simulink model "reaction_pendulum_LQR_LETSEEWHATHAPPENSGUYS"  (R2021b)
settings: Solver=FixedStepDiscrete  StartTime=0.0  StopTime=inf  FixedStep=h  RelTol=1e-3  EnableMultiTasking=on
PreLoadFcn:
  | warning('off','MATLAB:dispatcher:InexactMatch');
InitFcn:
  | hwinit
values from neighbouring files (symbols this model uses):
  A = [0.989609173212  0  0; 0  1  0.01; -0.000301949872013  -0.0950246262215  0.997224421049]    [MATRICES.mat]    (also in SS_11_5.mat = [0.9904  0  0; 0  1  0.01; -9e-05  -0.033262024  0.99812133]; WEAREGOINGHOMEMATRICES.mat = [0.989609173212  0  0; 0  1  0.01; 0.000423899858033  -0.095; current_SS.mat = [0.989609173212  0  0; 0  1  0.01; -9.34612180115e-05  -0.02; dynamicUpdateModel.m = [1.000494318995348 0.010001647563961 2.391143629140888e-07)
  Aeq = [Aeq; Ax0]    [Manual_MPC_Companion.m]    (also in Manual_MPC_Companion_THURSDAY.m = zeros(n * Np, n_total))
  B = [4.20519003073 0 0]    [MATRICES.mat]    (also in SS_11_5.mat = [4.1334 0 0]; current_SS.mat; dynamicUpdateModel.m = [-1.828407620987413e-04; full_dynamics.m = dsys.B)
  beq = zeros(n_total,1)    [Manual_MPC_Companion.m]    (also in Manual_MPC_Companion_THURSDAY.m = zeros(n * Np, 1))
  C = [1 0 0; 0 1 0]    [MeasModel.m]    (also in SS_11_5.mat = [1  0  0; 0  1  0]; current_SS.mat = [1  0  0; 0  1  0]; full_dynamics.m = dsys.C; full_system_ID.m = sys_est.C)
  H = diag([kron(ones(1,Np), Q) kron(ones(1,Np), R)])    [Manual_MPC_Companion.m]    (also in Manual_MPC_Companion_THURSDAY.m = blkdiag(Qbar, Rbar))
  h = 0.01    [SS_11_5.mat]    (also in hwinit.m)
  lb = [-1e6*ones(nx_total,1); -ones(m*Np,1)]    [Manual_MPC_Companion.m]    (also in Manual_MPC_Companion_THURSDAY.m = [-1e6*ones(nx_total, 1); -ones(nu_total, 1)])
  ub = [1e6*ones(nx_total,1); ones(m*Np,1)]    [Manual_MPC_Companion.m]    (also in Manual_MPC_Companion_THURSDAY.m = [ 1e6*ones(nx_total, 1);  ones(nu_total, 1)])
undefined symbols (not defined in the file or in its folder): cThresh, Discrete, E_ref, g_eff, K, K_bottom, k_e, magnitude, Time
libraries: simulink x3, ctrlSharedLib x2, mpclib x1
settings Model: SimulationMode=external  ExtModeTrigDuration=100000  Creator=user  LastModifiedBy=suray
settings DataIOCC: SaveFormat=Array  SignalLoggingSaveFormat=ModelDataLogs  SaveOutput=off  SignalLogging=off  DSMLogging=off  SaveTime=off  ReturnWorkspaceOutputs=off
settings OptimizationCC: ExpressionDepthLimit=2147483647  LifeSpan=inf
settings DebuggingCC: UnderspecifiedInitializationDetection=Classic  MergeDetectMultiDrivingBlocksExec=none  SolverPrmCheckMsg=warning  FcnCallInpInsideContextMsg=warning  StateNameClashWarn=warning  SFUnexpectedBacktrackingDiag=warning  SFNoUnconditionalDefaultTransitionDiag=warning  SFExecutionAtInitializationDiag=none  ArithmeticOperatorsInVariantConditions=warning
settings HardwareCC: ProdBitPerPointer=32  ProdBitPerSizeT=32  ProdBitPerPtrDiffT=32  ProdLargestAtomicFloat=None  ProdIntDivRoundTo=Undefined  ProdEndianess=Unspecified  ProdWordSize=32  ProdHWDeviceType=32-bit Generic
settings ModelReferenceCC: PropagateSignalLabelsOutOfModel=off
settings SFSimCC: SimUseLocalCustomCode=off  CustomCodeUndefinedFunction=UseInterfaceOnly
settings RTWCC: Description=rpend RTDAC/USB2 (Visual C/C++)  SystemTargetFile=rtcon_rpend_usb2.tlc  TemplateMakefile=rtcon_rpend_vc_usb2_x64.tmf  RTWUseLocalCustomCode=off
settings CodeAppCC: StateflowObjectComments=on
settings STFCustomTargetCC: ModelReferenceCompliant=off  CombineOutputUpdateFcns=on  MatFileLogging=on  GRTInterface=off  SystemTargetFile=rtcon_rpend_usb2.tlc
settings GRTTargetCC: TargetLangStandard=C89/C90 (ANSI)  ModelReferenceCompliant=off  ParMdlRefBuildCompliant=off  CompOptLevelCompliant=off  ConcurrentExecutionCompliant=off  CPPClassGenCompliant=off  UseToolchainInfoCompliant=off  ExtMode=on  ExtModeMexFile=rtcon_ext_comm
settings ConfigComp: CovMetricSettings=dw  CovSaveCumulativeToWorkspaceVar=on  CovSaveSingleToWorkspaceVar=on  CovExternalEMLEnable=off  CovSFcnEnable=off

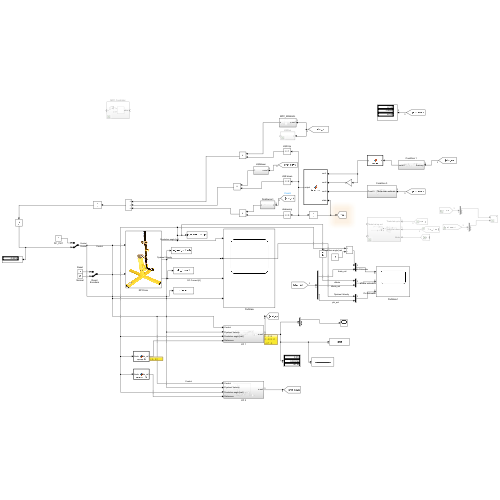
[thumbnail: Simulink's stored preview of the top-level diagram]
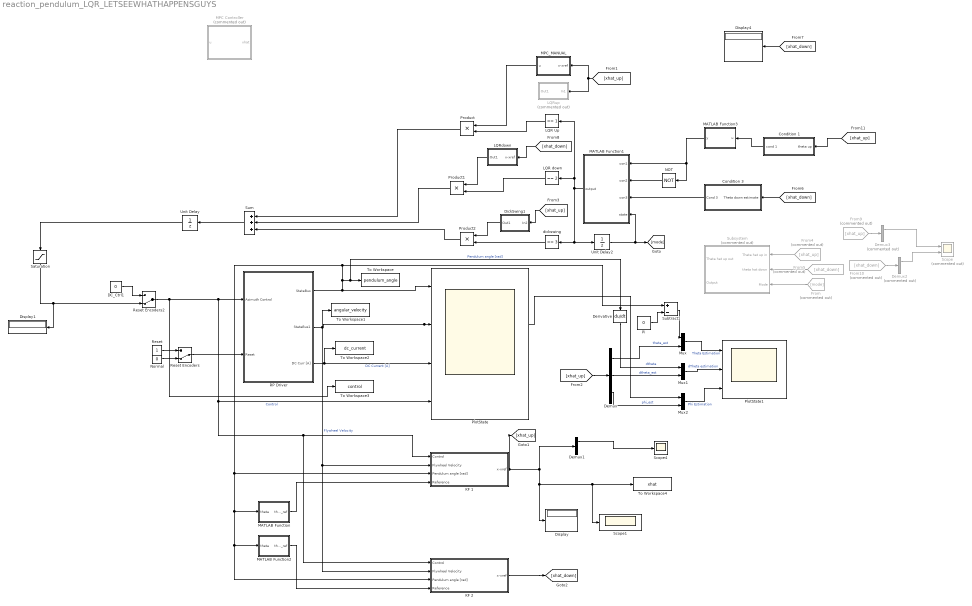
== system reaction_pendulum_LQR_LETSEEWHATHAPPENSGUYS ==
  Condition 1 : Subsystem
  Condition 3 : Subsystem
  DC_Ctrl1 : Constant  Value=0
  Demux : Demux  Outputs=3
  Demux1 : Demux  Outputs=3
  Demux2 : Demux  Commented=on  Outputs=3
  Demux3 : Demux  Commented=on  Outputs=3
  Derivative : Derivative
  DickSwing1 : Subsystem
  Display : Display
  Display1 : Display
  Display4 : Display
  From : From  Commented=on  GotoTag=mode
  From10 : From  Commented=on  GotoTag=xhat_down
  From4 : From  Commented=on  GotoTag=xhat_up
  From5 : From  Commented=on  GotoTag=xhat_down
  From9 : From  Commented=on  GotoTag=xhat_up
  KF 1 : Subsystem
  KF 2 : Subsystem
  LQR Up : simulink/Logic and Bit Operations/Compare To Constant  relop===  const=1  OutDataTypeStr=uint8
  LQR down : simulink/Logic and Bit Operations/Compare To Constant  relop===  const=2  OutDataTypeStr=uint8
  LQRdown : Subsystem
  LQRup : Subsystem  Commented=on
  MATLAB Function : MATLAB Function  TreatAsAtomicUnit=on
  MATLAB Function1 : MATLAB Function  TreatAsAtomicUnit=on
  MATLAB Function2 : MATLAB Function  TreatAsAtomicUnit=on
  MATLAB Function3 : MATLAB Function  TreatAsAtomicUnit=on
  MPC Controller : Subsystem  Commented=on
  MPC_MANUAL : Subsystem
  Mux : Mux  Inputs=2
  Mux1 : Mux  Inputs=2
  Mux2 : Mux  Inputs=2
  NOT : Logic  Operator=NOT  IconShape=distinctive  AllPortsSameDT=off  OutDataTypeStr=boolean
  Normal : Constant  Value=0
  Pi : Constant  Value=0  OutDataTypeStr=Inherit: Inherit via back propagation
  PlotState : Scope  NumInputPorts=4
  PlotState1 : Scope  NumInputPorts=3
  Product : Product
  Product1 : Product
  Product2 : Product
  RP Driver : Subsystem
      mask Display: image(imread('rwp.JPG'))
  Reset : Constant
  Reset Encoders : ManualSwitch  CurrentSetting=0
  Reset Encoders2 : ManualSwitch  CurrentSetting=0
  Saturation : Saturate  UpperLimit=1  LowerLimit=-1
  Scope : Scope  Commented=on  NumInputPorts=2
  Scope1 : Scope
  Scope4 : Scope
  Subsystem : Subsystem  Commented=on
  Subtract1 : Sum  Inputs=+-
  Sum : Sum  Inputs=+++
  To Workspace : ToWorkspace  VariableName=pendulum_angle  SaveFormat=Timeseries  SampleTime=-1
  To Workspace1 : ToWorkspace  VariableName=angular_velocity  SaveFormat=Timeseries  SampleTime=-1
  To Workspace2 : ToWorkspace  VariableName=dc_current  SaveFormat=Timeseries  SampleTime=-1
  To Workspace3 : ToWorkspace  VariableName=control  SaveFormat=Timeseries  SampleTime=-1
  To Workspace4 : ToWorkspace  VariableName=xhat  SaveFormat=Timeseries  SampleTime=-1
  Unit Delay : UnitDelay  SampleTime=0.01
  Unit Delay2 : UnitDelay  InitialCondition=3  SampleTime=h  HasFrameUpgradeWarning=on
  dickswing : simulink/Logic and Bit Operations/Compare To Constant  relop===  const=3  OutDataTypeStr=uint8
  wires:
  Normal/1 -> Reset Encoders/2
  Reset/1 -> Reset Encoders/1
  Reset Encoders/1 -> RP Driver/2(Reset)
  RP Driver/3(DC Curr [A]) -> To Workspace2/1, PlotState/3  "DC Current [A]"
  RP Driver/1(StateBus) -> Derivative/1, To Workspace/1, KF 1/3(Pendulum angle [rad]), KF 2/3(Pendulum angle [rad]), MATLAB Function2/1(theta), MATLAB Function/1(theta), Subtract1/1, PlotState/1  "Pendulum angle [rad]"
  Demux/3 -> Mux2/2  "phi_est"
  Demux/2 -> Mux1/2  "dtheta_est"
  Demux/1 -> Mux/2  "theta_est"
  Derivative/1 -> Mux1/1  "dtheta"
  Mux/1 -> PlotState1/1  "Theta Estimation"
  Mux1/1 -> PlotState1/2  "dTheta estimation"
  Mux2/1 -> PlotState1/3  "Phi Estimation"
  Saturation/1 -> Display1/1, Reset Encoders2/2
  DC_Ctrl1/1 -> Reset Encoders2/1
  Pi/1 -> Subtract1/2
  Subtract1/1 -> Mux/1
  Unit Delay/1 -> Saturation/1
  Unit Delay2/1 -> MATLAB Function1/4(state), [mode]
  LQR Up/1 -> Product/2
  LQR down/1 -> Product1/2
  MATLAB Function1/1(output) -> dickswing/1, Unit Delay2/1, LQR Up/1, LQR down/1
  dickswing/1 -> Product2/2
  Product/1 -> Sum/1
  Product1/1 -> Sum/2
  Product2/1 -> Sum/3
  NOT/1 -> MATLAB Function1/2(con2)
  DickSwing1/1(Out1) -> Product2/1
  LQRdown/1(Out1) -> Product1/1
  Reset Encoders2/1 -> KF 1/1(Control), KF 2/1(Control), PlotState/4, RP Driver/1(Azimuth Control), To Workspace3/1  "Control"
  RP Driver/2(StateBus1) -> Mux2/1, PlotState/2, To Workspace1/1, KF 2/2(Flywheel Velocity), KF 1/2(Flywheel Velocity)  "Flywheel Velocity"
  MATLAB Function2/1(theta_ref) -> KF 2/4(Reference)
  MATLAB Function/1(theta_ref) -> KF 1/4(Reference)
  KF 2/1(x-xref) -> [xhat_down]
  Sum/1 -> Unit Delay/1
  Demux1/1 -> Scope4/1
  KF 1/1(x-xref) -> [xhat_up], Display/1, Scope1/1, To Workspace4/1, Demux1/1
  From/1 -> Subsystem/3(Mode)
  Condition 3/1(Cond 3) -> MATLAB Function1/3(con3)
  Condition 1/1(cond 1) -> MATLAB Function3/1(u)
  [xhat_up] -> MPC_MANUAL/1(x-xref), LQRup/1(In1)
  [xhat_up] -> Demux/1
  [xhat_up] -> DickSwing1/1(In2)
  From4/1 -> Subsystem/1(Theta hat up in)
  From5/1 -> Subsystem/2(theta hat down)
  [xhat_down] -> Condition 3/1(Theta down estimate)
  [xhat_down] -> Display4/1
  [xhat_down] -> LQRdown/1(x-xref)
  From9/1 -> Demux3/1
  Demux3/1 -> Scope/1
  From10/1 -> Demux2/1
  Demux2/1 -> Scope/2
  MATLAB Function3/1(y) -> MATLAB Function1/1(con1), NOT/1
  [xhat_up] -> Condition 1/1(theta up)
  MPC_MANUAL/1(u) -> Product/1

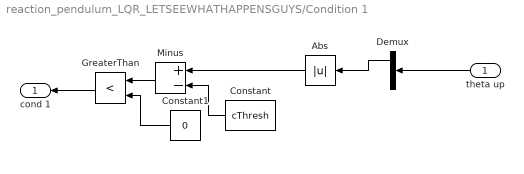
== system reaction_pendulum_LQR_LETSEEWHATHAPPENSGUYS/Condition 1 ==
  theta up : Inport
  Abs : Abs
  Constant : Constant  Value=cThresh
  Constant1 : Constant  Value=0
  Demux : Demux  Outputs=3
  GreaterThan : RelationalOperator  Operator=<  OutDataTypeStr=boolean  RndMeth=Simplest
  Minus : Sum  Inputs=+-
  cond 1 : Outport
  wires:
  Constant1/1 -> GreaterThan/2
  theta up/1 -> Demux/1
  Constant/1 -> Minus/2
  Minus/1 -> GreaterThan/1
  GreaterThan/1 -> cond 1/1
  Abs/1 -> Minus/1
  Demux/1 -> Abs/1

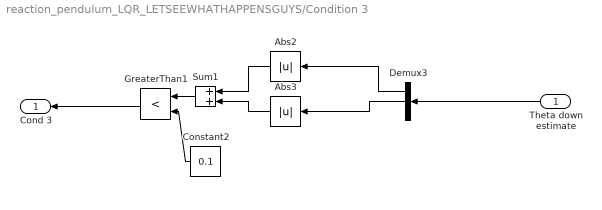
== system reaction_pendulum_LQR_LETSEEWHATHAPPENSGUYS/Condition 3 ==
  Theta down estimate : Inport
  Abs2 : Abs
  Abs3 : Abs
  Constant2 : Constant  Value=0.1
  Demux3 : Demux  Outputs=3
  GreaterThan1 : RelationalOperator  Operator=<  OutDataTypeStr=boolean  RndMeth=Simplest
  Sum1 : Sum
  Cond 3 : Outport
  wires:
  Demux3/2 -> Abs3/1
  Demux3/1 -> Abs2/1
  Abs2/1 -> Sum1/1
  GreaterThan1/1 -> Cond 3/1
  Constant2/1 -> GreaterThan1/2
  Sum1/1 -> GreaterThan1/1
  Abs3/1 -> Sum1/2
  Theta down estimate/1 -> Demux3/1

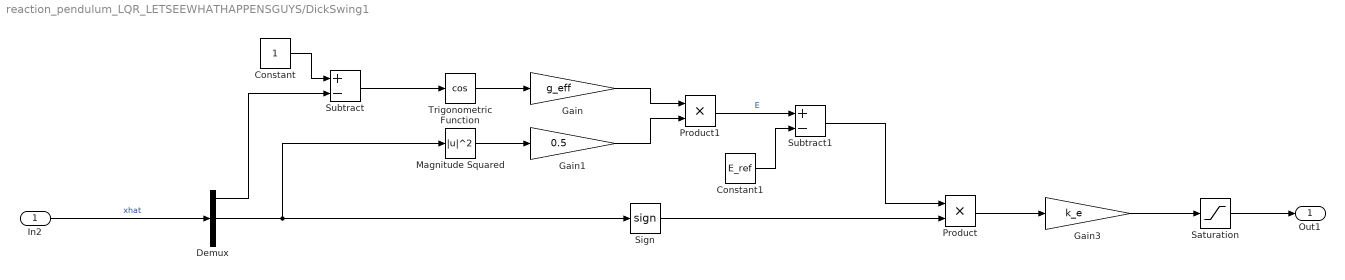
== system reaction_pendulum_LQR_LETSEEWHATHAPPENSGUYS/DickSwing1 ==
  In2 : Inport
  Constant : Constant
  Constant1 : Constant  Value=E_ref
  Demux : Demux  Outputs=3
  Gain : Gain  Gain=g_eff
  Gain1 : Gain  Gain=0.5
  Gain3 : Gain  Gain=k_e
  Magnitude Squared : Math  Operator=magnitude^2  SaturateOnIntegerOverflow=on
  Product : Product
  Product1 : Product
  Saturation : Saturate  UpperLimit=0.75  LowerLimit=-0.75
  Sign : Signum
  Subtract : Sum  Inputs=+-
  Subtract1 : Sum  Inputs=+-
  Trigonometric Function : Trigonometry  Operator=cos
  Out1 : Outport
  wires:
  In2/1 -> Demux/1  "xhat"
  Trigonometric Function/1 -> Gain/1
  Magnitude Squared/1 -> Gain1/1
  Gain/1 -> Product1/1
  Gain1/1 -> Product1/2
  Constant/1 -> Subtract/1
  Subtract/1 -> Trigonometric Function/1
  Demux/1 -> Subtract/2
  Sign/1 -> Product/2
  Product1/1 -> Subtract1/1  "E"
  Constant1/1 -> Subtract1/2
  Subtract1/1 -> Product/1
  Product/1 -> Gain3/1
  Gain3/1 -> Saturation/1
  Demux/2 -> Magnitude Squared/1, Sign/1
  Saturation/1 -> Out1/1

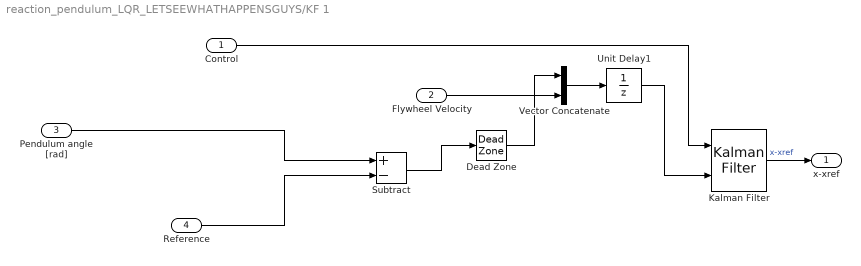
== system reaction_pendulum_LQR_LETSEEWHATHAPPENSGUYS/KF 1 ==
  Control : Inport
  Flywheel Velocity : Inport  Port=2
  Pendulum angle [rad] : Inport  Port=3
  Reference : Inport  Port=4
  Dead Zone : DeadZone  LowerValue=0  UpperValue=0.0  SaturateOnIntegerOverflow=on
  Kalman Filter : ctrlSharedLib/Kalman Filter  TimeDomain=Discrete-Time  UseCurrentEstimator=on  ModelSource=Individual A, B, C, D matrices  ModelSourceVariable=ss(0.95,1,1,0,1)  A=A  B=B  C=C  D=[0;0]  NumberOfStates=1  NumberOfInputs=1  NumberOfOutputs=1  InitialEstimateSource=Dialog  X0=0  P0=10  UseK=off  UseGH=off  NumberOfProcessNoiseInputs=1  G=1  TimeInvariantG=on  H=0  TimeInvariantH=on  Q=diag([0.00001 0.05 0.0001])  TimeInvariantQ=on  R=diag([0.0001 0.01])  TimeInvariantR=on  N=0  TimeInvariantN=on  AddInputPort=on  AddEnablePort=off  OutputEstimatedY=off  OutputP=off  Ts=-1
  Subtract : Sum  Inputs=+-
  Unit Delay1 : UnitDelay  SampleTime=0.01
  Vector Concatenate : Concatenate
  x-xref : Outport
  wires:
  Kalman Filter/1 -> x-xref/1  "x-xref"
  Subtract/1 -> Dead Zone/1
  Reference/1 -> Subtract/2
  Dead Zone/1 -> Vector Concatenate/1
  Flywheel Velocity/1 -> Vector Concatenate/2
  Unit Delay1/1 -> Kalman Filter/2
  Vector Concatenate/1 -> Unit Delay1/1
  Pendulum angle [rad]/1 -> Subtract/1
  Control/1 -> Kalman Filter/1

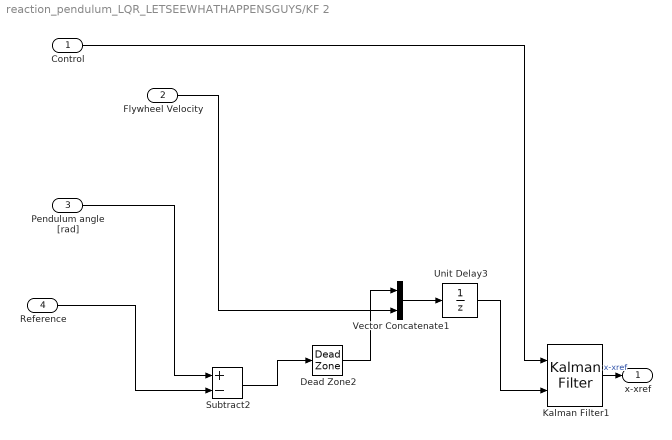
== system reaction_pendulum_LQR_LETSEEWHATHAPPENSGUYS/KF 2 ==
  Control : Inport
  Flywheel Velocity : Inport  Port=2
  Pendulum angle [rad] : Inport  Port=3
  Reference : Inport  Port=4
  Dead Zone2 : DeadZone  LowerValue=0  UpperValue=0.0  SaturateOnIntegerOverflow=on
  Kalman Filter1 : ctrlSharedLib/Kalman Filter  TimeDomain=Discrete-Time  UseCurrentEstimator=on  ModelSource=Individual A, B, C, D matrices  ModelSourceVariable=ss(0.95,1,1,0,1)  A=A  B=B  C=C  D=[0;0]  NumberOfStates=1  NumberOfInputs=1  NumberOfOutputs=1  InitialEstimateSource=Dialog  X0=0  P0=10  UseK=off  UseGH=off  NumberOfProcessNoiseInputs=1  G=1  TimeInvariantG=on  H=0  TimeInvariantH=on  Q=diag([0.00001 0.05 0.0001])  TimeInvariantQ=on  R=diag([0.0001 0.01])  TimeInvariantR=on  N=0  TimeInvariantN=on  AddInputPort=on  AddEnablePort=off  OutputEstimatedY=off  OutputP=off  Ts=-1
  Subtract2 : Sum  Inputs=+-
  Unit Delay3 : UnitDelay  SampleTime=0.01
  Vector Concatenate1 : Concatenate
  x-xref : Outport
  wires:
  Unit Delay3/1 -> Kalman Filter1/2
  Pendulum angle [rad]/1 -> Subtract2/1
  Reference/1 -> Subtract2/2
  Dead Zone2/1 -> Vector Concatenate1/1
  Control/1 -> Kalman Filter1/1
  Subtract2/1 -> Dead Zone2/1
  Vector Concatenate1/1 -> Unit Delay3/1
  Flywheel Velocity/1 -> Vector Concatenate1/2
  Kalman Filter1/1 -> x-xref/1  "x-xref"

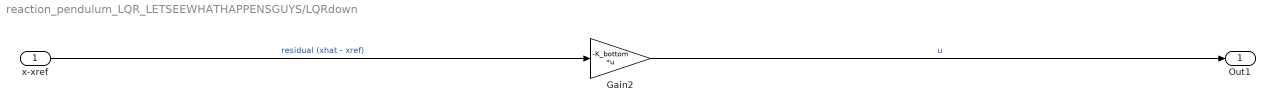
== system reaction_pendulum_LQR_LETSEEWHATHAPPENSGUYS/LQRdown ==
  x-xref : Inport
  Gain2 : Gain  Gain=-K_bottom  Multiplication=Matrix(K*u) (u vector)
  Out1 : Outport
  wires:
  x-xref/1 -> Gain2/1  "residual (xhat - xref)"
  Gain2/1 -> Out1/1  "u"

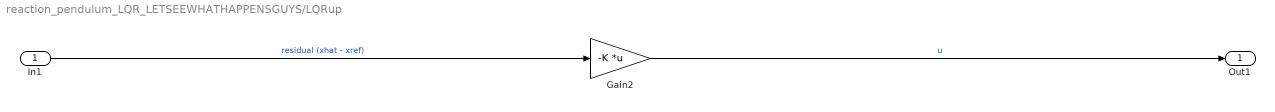
== system reaction_pendulum_LQR_LETSEEWHATHAPPENSGUYS/LQRup ==
  In1 : Inport
  Gain2 : Gain  Gain=-K  Multiplication=Matrix(K*u) (u vector)
  Out1 : Outport
  wires:
  In1/1 -> Gain2/1  "residual (xhat - xref)"
  Gain2/1 -> Out1/1  "u"

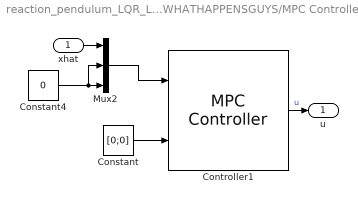
== system reaction_pendulum_LQR_LETSEEWHATHAPPENSGUYS/MPC Controller ==
  xhat : Inport
  Constant : Constant  Value=[0;0]
  Constant4 : Constant  Value=0
  Controller1 : mpclib/MPC Controller  SCDEnableBlockLinearizationSpecification=on  mpcobj=MPC_controller  is_multiple=0  enable_value=0  return_u0=off  updateMPCinCallerWorkspace=on  md_inport=off  mv_inport=off  uref_inport=off  return_cost=off  return_mvseq=off  return_qpstatus=off  return_xseq=off  return_state=off  return_ovseq=off  state_inport=on  umin_inport=off  umax_inport=off  ymin_inport=off  ymax_inport=off  cc_inport=off  ywt_inport=off  uwt_inport=off  duwt_inport=off  rhoeps_inport=off  pm_inport=off  MaximumP=10  HorizonChoice=FixedHorizon  n_ts=0.01  n_p=30  n_mv=1  n_md=0  n_ud=0  n_mo=2  n_uo=0  BlockDataType=double  SampleTimeInherited=off  switch_inport=off
  Mux2 : Mux  Inputs=3
  u : Outport
  wires:
  Controller1/1 -> u/1  "u"
  xhat/1 -> Mux2/1
  Constant4/1 -> Mux2/3, Mux2/2
  Mux2/1 -> Controller1/1
  Constant/1 -> Controller1/2

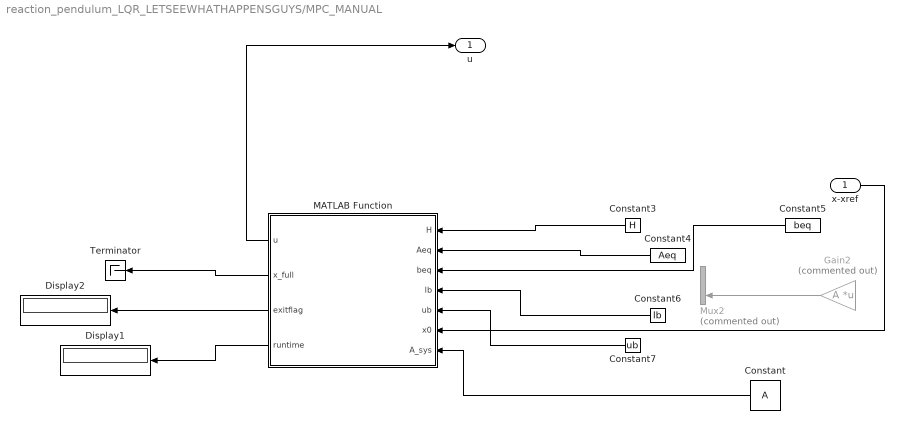
== system reaction_pendulum_LQR_LETSEEWHATHAPPENSGUYS/MPC_MANUAL ==
  x-xref : Inport
  Constant : Constant  Value=A  VectorParams1D=off
  Constant3 : Constant  Value=H
  Constant4 : Constant  Value=Aeq
  Constant5 : Constant  Value=beq
  Constant6 : Constant  Value=lb
  Constant7 : Constant  Value=ub
  Display1 : Display
  Display2 : Display
  Gain2 : Gain  Commented=on  Gain=A  Multiplication=Matrix(K*u) (u vector)
  MATLAB Function : MATLAB Function  TreatAsAtomicUnit=on
  Mux2 : Mux  Commented=on  Inputs=2
  Terminator : Terminator
  u : Outport
  wires:
  Constant3/1 -> MATLAB Function/1(H)
  Constant4/1 -> MATLAB Function/2(Aeq)
  Constant5/1 -> MATLAB Function/3(beq)
  Constant6/1 -> MATLAB Function/4(lb)
  MATLAB Function/3(exitflag) -> Display2/1
  Gain2/1 -> Mux2/2
  Constant7/1 -> MATLAB Function/5(ub)
  MATLAB Function/4(runtime) -> Display1/1
  MATLAB Function/2(x_full) -> Terminator/1
  x-xref/1 -> MATLAB Function/6(x0)
  MATLAB Function/1(u) -> u/1
  Constant/1 -> MATLAB Function/7(A_sys)

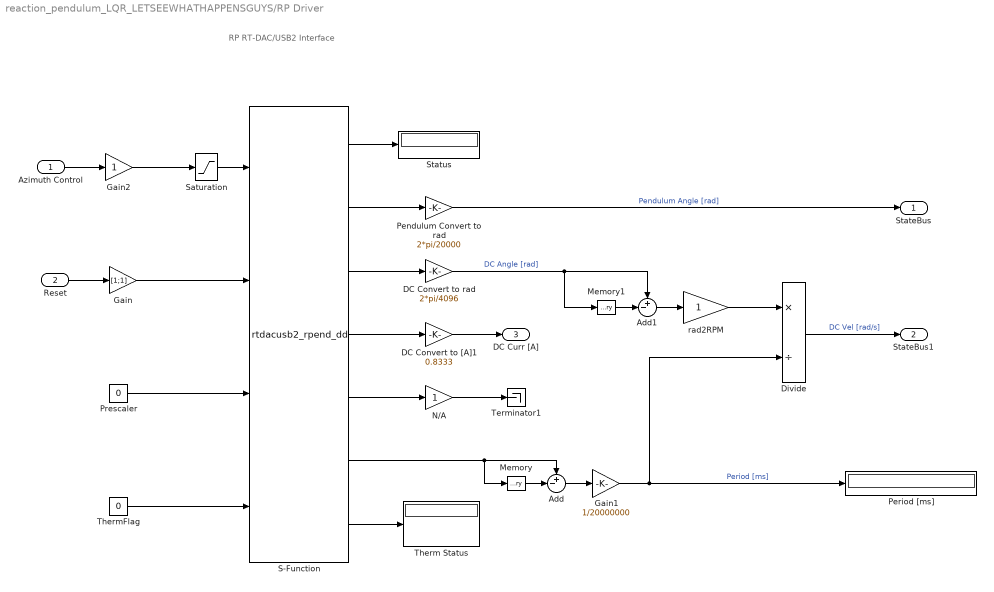
== system reaction_pendulum_LQR_LETSEEWHATHAPPENSGUYS/RP Driver ==
  note: RP RT-DAC/USB2
      | Interface
  Azimuth Control : Inport
  Reset : Inport  Port=2
  Add : Sum  Inputs=+-|
  Add1 : Sum  Inputs=+-|
  DC Convert to [A]1 : Gain  Gain=0.8333  SaturateOnIntegerOverflow=on  OutDataTypeStr=Inherit: Same as input  ParamDataTypeStr=Inherit: Same as input
  DC Convert to rad : Gain  Gain=2*pi/4096  SaturateOnIntegerOverflow=on  OutDataTypeStr=Inherit: Same as input  ParamDataTypeStr=Inherit: Same as input
  Divide : Product  Inputs=*/
  Gain : Gain  Gain=[1;1]
  Gain1 : Gain  Gain=1/20000000
  Gain2 : Gain
  Memory : Memory
  Memory1 : Memory
  N/A : Gain  SaturateOnIntegerOverflow=on  OutDataTypeStr=Inherit: Same as input  ParamDataTypeStr=Inherit: Same as input
  Pendulum Convert to rad : Gain  Gain=2*pi/20000  SaturateOnIntegerOverflow=on  OutDataTypeStr=Inherit: Same as input  ParamDataTypeStr=Inherit: Same as input
  Period [ms] : Display
  Prescaler : Constant  Value=0
  S-Function : S-Function  FunctionName=rtdacusb2_rpend_dd  Parameters=1, h  SFunctionDeploymentMode=off  EnableBusSupport=off
  Saturation : Saturate  UpperLimit=1  LowerLimit=-1
  Status : Display
  Terminator1 : Terminator
  Therm Status : Display
  ThermFlag : Constant  Value=0
  rad2RPM : Gain  SaturateOnIntegerOverflow=on  OutDataTypeStr=Inherit: Same as input  ParamDataTypeStr=Inherit: Same as input
  StateBus : Outport  VectorParamsAs1DForOutWhenUnconnected=off
  StateBus1 : Outport  Port=2  VectorParamsAs1DForOutWhenUnconnected=off
  DC Curr [A] : Outport  Port=3  VectorParamsAs1DForOutWhenUnconnected=off
  wires:
  S-Function/7 -> Therm Status/1
  S-Function/5 -> N/A/1
  S-Function/4 -> DC Convert to [A]1/1
  ThermFlag/1 -> S-Function/4
  Prescaler/1 -> S-Function/3
  Gain/1 -> S-Function/2
  DC Convert to [A]1/1 -> DC Curr [A]/1
  Divide/1 -> StateBus1/1  "DC Vel [rad/s]"
  rad2RPM/1 -> Divide/1
  Add1/1 -> rad2RPM/1
  Memory1/1 -> Add1/2
  N/A/1 -> Terminator1/1
  S-Function/6 -> Add/1, Memory/1
  Gain2/1 -> Saturation/1
  Gain1/1 -> Period [ms]/1, Divide/2  "Period [ms]"
  Add/1 -> Gain1/1
  Memory/1 -> Add/2
  DC Convert to rad/1 -> Add1/1, Memory1/1  "DC Angle [rad]"
  S-Function/3 -> DC Convert to rad/1
  Pendulum Convert to rad/1 -> StateBus/1  "Pendulum Angle [rad]"
  S-Function/2 -> Pendulum Convert to rad/1
  S-Function/1 -> Status/1
  Saturation/1 -> S-Function/1
  Reset/1 -> Gain/1
  Azimuth Control/1 -> Gain2/1

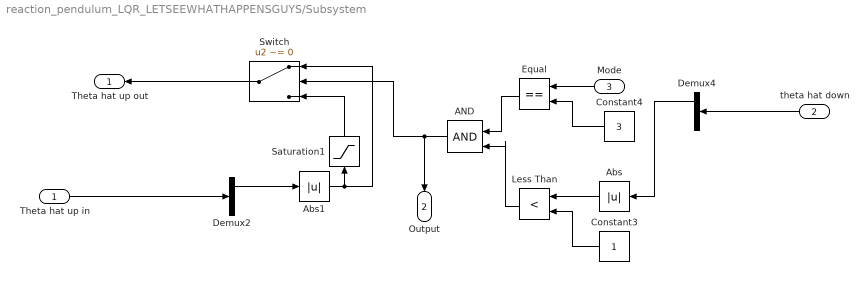
== system reaction_pendulum_LQR_LETSEEWHATHAPPENSGUYS/Subsystem ==
  Theta hat up in : Inport
  theta hat down : Inport  Port=2
  Mode : Inport  Port=3
  AND : Logic  IconShape=distinctive  AllPortsSameDT=off  OutDataTypeStr=boolean
  Abs : Abs
  Abs1 : Abs
  Constant3 : Constant
  Constant4 : Constant  Value=3
  Demux2 : Demux  Outputs=3
  Demux4 : Demux  Outputs=3
  Equal : RelationalOperator  Operator===  OutDataTypeStr=boolean  RndMeth=Simplest
  Less Than : RelationalOperator  Operator=<  OutDataTypeStr=boolean  RndMeth=Simplest
  Saturation1 : Saturate  UpperLimit=inf  LowerLimit=cThresh + 1e-6
  Switch : Switch  Criteria=u2 ~= 0
  Theta hat up out : Outport
  Output : Outport  Port=2
  wires:
  Abs/1 -> Less Than/1
  Abs1/1 -> Saturation1/1, Switch/1
  Demux2/1 -> Abs1/1
  Equal/1 -> AND/1
  Constant4/1 -> Equal/2
  Constant3/1 -> Less Than/2
  Mode/1 -> Equal/1
  Less Than/1 -> AND/2
  Demux4/1 -> Abs/1
  AND/1 -> Output/1, Switch/2
  Saturation1/1 -> Switch/3
  theta hat down/1 -> Demux4/1
  Switch/1 -> Theta hat up out/1
  Theta hat up in/1 -> Demux2/1

== matlab function reaction_pendulum_LQR_LETSEEWHATHAPPENSGUYS/MPC_MANUAL/MATLAB Function ==
  data: u output size=1; H input; Aeq input; beq input; lb input; ub input; x_full output; exitflag output; runtime output; x0 input; A_sys input
% function [u, x_full, exitflag, runtime] = MPC_short(H, A, b, lb, ub)
% tic
% f  = zeros(size(H,1),1);
% Aineq = zeros(0,size(H,1));
% bineq = zeros(0,1);
% x0 = zeros(size(H,1),1);
% T = size(H,1)/4; % n + m = 4
% 
% opts = optimoptions('quadprog', ...
%     'Algorithm','active-set');
% [x_full, fval, exitflag, output] = quadprog(H, f, Aineq, bineq, A, b, lb, ub, x0, opts);
% u = x_full(3*T+1); % u1
% runtime = toc;

function [u, x_full, exitflag, runtime] = MPC_short(H, Aeq, beq, lb, ub, x0, A_sys)
tic

n = size(A_sys, 1);
T = size(H, 1) / 4;  % Np, since n+m = 4

% Inject current state into the last n rows of beq
beq(end-n+1 : end) = A_sys * x0;

f      = zeros(size(H, 1), 1);
Aineq  = zeros(0, size(H, 1));
bineq  = zeros(0, 1);
x0_qp  = zeros(size(H, 1), 1);

opts = optimoptions('quadprog', 'Algorithm', 'active-set');

[x_full, ~, exitflag, ~] = quadprog(H, f, Aineq, bineq, Aeq, beq, lb, ub, x0_qp, opts);

u = x_full(3*T + 1);  % first control input u_1
runtime = toc;
end

== matlab function reaction_pendulum_LQR_LETSEEWHATHAPPENSGUYS/MATLAB Function ==
  data: theta input; theta_ref output
function theta_ref = nearestPi(theta)
k = round((theta-pi)/(2*pi));
theta_ref = (2*k + 1)*pi;
end

== matlab function reaction_pendulum_LQR_LETSEEWHATHAPPENSGUYS/MATLAB Function1 ==
  data: con1 input; output output; con2 input; con3 input; state input
function output = twswitch(con1, con2, con3, state)
output = 3;
action = 0;
switch state
    case 1
        if con2
            output = 2;
            action = 1;
        end
    case 2
        if con3
            output = 3;
            action = 1;
        end
    case 3
        if con1
            output = 1;
            action = 1;
        end
end
if not(action)
    output = state;
end

== matlab function reaction_pendulum_LQR_LETSEEWHATHAPPENSGUYS/MATLAB Function2 ==
  data: theta input; theta_ref output
function theta_ref = nearest2Pi(theta)
k = round((theta)/(2*pi));
theta_ref = 2*k*pi;
end

== matlab function reaction_pendulum_LQR_LETSEEWHATHAPPENSGUYS/MATLAB Function3 ==
  data: u input; y output
function y = delay(u)

N = 3; % 3 consecutive samples

persistent count

if isempty(count)
    count = 0;
end

if u
    count = count + 1;
else
    count = 0;
end

y = count >= N;
